simulink model "Target_Control_System"  (R2021b)
settings: Solver=FixedStepDiscrete  StartTime=0.0  StopTime=5  RelTol=1e-3
PreLoadFcn:
  | RTWConfigurationCB('preloadfcn', bdroot);
PostLoadFcn:
  | load('configuration/data_struct.mat');
  | load('configuration/fluxMaps_propMotor.mat');
  | load('configuration/parameterInit_PROP.mat');
  | load('configuration/parameterInit_PUMP.mat');
  | load('configuration/parameterInit_PITCH.mat');
  | load('configuration/parameterInit_TILT.mat');
  | %load('configuration/base_workspace_signal_definition.mat');
  | %load('resolvedatastores_to_baseworkspace_for_faster_simulation.mat');
model workspace (MAT data in the model file):
  SIMULATION_OPTIONS : Simulink.Parameter (value not decoded)
  TARGET_CODE_GEN : Simulink.Parameter (value not decoded)
  TCS_SAMPLE_FREQ_HZ : Simulink.Parameter (value not decoded)
symbols that are objects in the model workspace (value not decoded): TARGET_CODE_GEN, TCS_SAMPLE_FREQ_HZ
undefined symbols (not defined in the file): A_DQ_REF_LPF_INIT__PITCH, A_DQ_REF_LPF_INIT__PROP, A_DQ_REF_LPF_INIT__PUMP, A_DQ_REF_LPF_INIT__TILT, A_OBSERVER_CONFIDENCE_INIT__PITCH, A_OBSERVER_CONFIDENCE_INIT__PROP, A_OBSERVER_CONFIDENCE_INIT__PUMP, A_OBSERVER_CONFIDENCE_INIT__TILT, ACTUATOR_MAX_ANGLE_TRIP__PITCH, ACTUATOR_MIN_ANGLE_TRIP__PITCH, ACTUATOR_POS_SENSOR_INV_DIRECTION__PITCH, ACTUATOR_POS_SENSOR_INV_DIRECTION__TILT, ACTUATOR_POS_SENSOR_OFFSET__PITCH, ACTUATOR_POS_SENSOR_OFFSET__TILT, ADC_scaler1_baseaddr_TILT, ADC_SCALER_FLOAT_TO_FIXPOINT_EXPANSION, ANGLE_ELEC_FROM_SENSOR_OFFSET_INIT__PITCH, ANGLE_ELEC_FROM_SENSOR_OFFSET_INIT__PROP, ANGLE_ELEC_FROM_SENSOR_OFFSET_INIT__PUMP, ANGLE_ELEC_FROM_SENSOR_OFFSET_INIT__TILT, AUTO_CLEAR_FAULTS_ENABLED__PITCH, AUTO_CLEAR_FAULTS_ENABLED__PROP, AUTO_CLEAR_FAULTS_ENABLED__PUMP, AUTO_CLEAR_FAULTS_ENABLED__TILT, AUTO_CLEAR_FAULTS_WAIT_TICKS__PITCH, AUTO_CLEAR_FAULTS_WAIT_TICKS__PROP, AUTO_CLEAR_FAULTS_WAIT_TICKS__PUMP, AUTO_CLEAR_FAULTS_WAIT_TICKS__TILT, AUTO_I_ZERO_IDLE_TICKS__PITCH, AUTO_I_ZERO_IDLE_TICKS__PROP, AUTO_I_ZERO_IDLE_TICKS__PUMP, AUTO_I_ZERO_IDLE_TICKS__TILT, AUTO_I_ZERO_OFFSET_IDC_THRESHOLD__PITCH, AUTO_I_ZERO_OFFSET_IDC_THRESHOLD__PROP, AUTO_I_ZERO_OFFSET_IDC_THRESHOLD__PUMP, AUTO_I_ZERO_OFFSET_IDC_THRESHOLD__TILT, AUTO_I_ZERO_OFFSET_IPH_THRESHOLD__PITCH, AUTO_I_ZERO_OFFSET_IPH_THRESHOLD__PROP, AUTO_I_ZERO_OFFSET_IPH_THRESHOLD__PUMP, AUTO_I_ZERO_OFFSET_IPH_THRESHOLD__TILT, AUTO_SENSORLESS_SWITCHOVER_DISABLE_OMEGA, AUTO_SENSORLESS_SWITCHOVER_ENABLE_OMEGA, AUTO_SENSORLESS_SWITCHOVER_MIN_CONFIDENCE, AUXILIARY_PROTECTION_UNIT_BASEADDR__TILT, blanking_max_error_omega_INIT_PITCH, blanking_max_error_omega_INIT_TILT, blanking_max_error_position_INIT_PITCH, blanking_max_error_position_INIT_TILT, BRUTE_START_I_Q_REF_RAMP_SPEED__PITCH, BRUTE_START_I_Q_REF_RAMP_SPEED__PROP, BRUTE_START_I_Q_REF_RAMP_SPEED__PUMP, BRUTE_START_I_Q_REF_RAMP_SPEED__TILT, CONTROL_LOOP_DT_INIT__PITCH, CONTROL_LOOP_DT_INIT__PROP, CONTROL_LOOP_DT_INIT__PUMP, CONTROL_LOOP_DT_INIT__TILT, CORRECTION_FILTER_SCALE__PITCH, CORRECTION_FILTER_SCALE__PROP, CORRECTION_FILTER_SCALE__PUMP, CORRECTION_FILTER_SCALE__TILT ... (+458)
libraries: simulink x178, Reusables_Lib x24
(part 10 of 47)

== system Target_Control_System/Target_Control_System/InterruptFunction/pitchMotor_isrTask/currentController/Current Controller ==
  Enable : EnablePort
  Add1 : Sum
  Data Store Read1 : DataStoreRead  DataStoreName=oPitch  DataStoreElements=oPitch.oIsr_.oState_.fId_  IndexOptions=Index vector (dialog)  Indices=1  OutputSizes=1
  Data Store Read10 : DataStoreRead  DataStoreName=oPitch  DataStoreElements=oPitch.oIsr_.oParam_.oPiDataId_.oParameter_.fIntMax_  IndexOptions=Index vector (dialog)  Indices=1  OutputSizes=1
  Data Store Read11 : DataStoreRead  DataStoreName=oPitch  DataStoreElements=oPitch.oIsr_.oParam_.oPiDataId_.oParameter_.fLoopDt_  IndexOptions=Index vector (dialog)  Indices=1  OutputSizes=1
  Data Store Read13 : DataStoreRead  DataStoreName=oPitch  DataStoreElements=oPitch.oIsr_.oIn_.fIqRefRampOut_  IndexOptions=Index vector (dialog)  Indices=1  OutputSizes=1
  Data Store Read14 : DataStoreRead  DataStoreName=oPitch  DataStoreElements=oPitch.oIsr_.oIn_.fIdRefFractionOfIq_  IndexOptions=Index vector (dialog)  Indices=1  OutputSizes=1
  Data Store Read15 : DataStoreRead  DataStoreName=oPitch  DataStoreElements=oPitch.oIsr_.oState_.fIq_  IndexOptions=Index vector (dialog)  Indices=1  OutputSizes=1
  Data Store Read16 : DataStoreRead  DataStoreName=oPitch  DataStoreElements=oPitch.oIsr_.oParam_.oPiDataIq_.oParameter_.fKp_  IndexOptions=Index vector (dialog)  Indices=1  OutputSizes=1
  Data Store Read17 : DataStoreRead  DataStoreName=oPitch  DataStoreElements=oPitch.oIsr_.oIn_.fOneOverUdc_  IndexOptions=Index vector (dialog)  Indices=1  OutputSizes=1
  Data Store Read18 : DataStoreRead  DataStoreName=oPitch  DataStoreElements=oPitch.oIsr_.oParam_.oPiDataIq_.oParameter_.fKi_  IndexOptions=Index vector (dialog)  Indices=1  OutputSizes=1
  Data Store Read19 : DataStoreRead  DataStoreName=oPitch  DataStoreElements=oPitch.oIsr_.oParam_.oPiDataIq_.oParameter_.fLoopDt_  IndexOptions=Index vector (dialog)  Indices=1  OutputSizes=1
  Data Store Read2 : DataStoreRead  DataStoreName=oPitch  DataStoreElements=oPitch.oIsr_.oParam_.oPiDataId_.oParameter_.fKp_  IndexOptions=Index vector (dialog)  Indices=1  OutputSizes=1
  Data Store Read20 : DataStoreRead  DataStoreName=oPitch  DataStoreElements=oPitch.oIsr_.oParam_.oPiDataIq_.oParameter_.fIntMax_  IndexOptions=Index vector (dialog)  Indices=1  OutputSizes=1
  Data Store Read21 : DataStoreRead  DataStoreName=oPitch  DataStoreElements=oPitch.oIsr_.oParam_.oPiDataIq_.oParameter_.fOutMax_  IndexOptions=Index vector (dialog)  Indices=1  OutputSizes=1
  Data Store Read22 : DataStoreRead  DataStoreName=oPitch  DataStoreElements=oPitch.oIsr_.oParam_.oPiDataIq_.oParameter_.fIntMin_  IndexOptions=Index vector (dialog)  Indices=1  OutputSizes=1
  Data Store Read23 : DataStoreRead  DataStoreName=oPitch  DataStoreElements=oPitch.oIsr_.oParam_.oPiDataIq_.oParameter_.fOutMin_  IndexOptions=Index vector (dialog)  Indices=1  OutputSizes=1
  Data Store Read24 : DataStoreRead  DataStoreName=oPitch  DataStoreElements=oPitch.oIsr_.oState_.fFluxMainMagnitudeLpf_  IndexOptions=Index vector (dialog)  Indices=1  OutputSizes=1
  Data Store Read25 : DataStoreRead  DataStoreName=oPitch  DataStoreElements=oPitch.oIsr_.oIn_.fFluxFeedforwardGainRampOut_  IndexOptions=Index vector (dialog)  Indices=1  OutputSizes=1
  Data Store Read26 : DataStoreRead  DataStoreName=oPitch  DataStoreElements=oPitch.oIsr_.oIn_.fOneOverUdc_  IndexOptions=Index vector (dialog)  Indices=1  OutputSizes=1
  Data Store Read27 : DataStoreRead  DataStoreName=oPitch  DataStoreElements=oPitch.oIsr_.oParam_.fMaximumVoltageVectorLengthSquared_  IndexOptions=Index vector (dialog)  Indices=1  OutputSizes=1
  Data Store Read29 : DataStoreRead  DataStoreName=mdl_pitch_fOmegaE  IndexOptions=Index vector (dialog)  Indices=1  OutputSizes=1
  Data Store Read3 : DataStoreRead  DataStoreName=oPitch  DataStoreElements=oPitch.oIsr_.oParam_.oPiDataId_.oParameter_.fKi_  IndexOptions=Index vector (dialog)  Indices=1  OutputSizes=1
  Data Store Read30 : DataStoreRead  DataStoreName=oPitch  DataStoreElements=oPitch.oIsr_.oParam_.oPiDataIq_.fState_  IndexOptions=Index vector (dialog)  Indices=1  OutputSizes=1
  Data Store Read31 : DataStoreRead  DataStoreName=oPitch  DataStoreElements=oPitch.oIsr_.oIn_.fIdRefRampOut_  IndexOptions=Index vector (dialog)  Indices=1  OutputSizes=1
  Data Store Read5 : DataStoreRead  DataStoreName=oPitch  DataStoreElements=oPitch.oIsr_.oIn_.fOneOverUdc_  IndexOptions=Index vector (dialog)  Indices=1  OutputSizes=1
  Data Store Read6 : DataStoreRead  DataStoreName=oPitch  DataStoreElements=oPitch.oIsr_.oParam_.oPiDataId_.fState_  IndexOptions=Index vector (dialog)  Indices=1  OutputSizes=1
  Data Store Read7 : DataStoreRead  DataStoreName=oPitch  DataStoreElements=oPitch.oIsr_.oParam_.oPiDataId_.oParameter_.fOutMin_  IndexOptions=Index vector (dialog)  Indices=1  OutputSizes=1
  Data Store Read8 : DataStoreRead  DataStoreName=oPitch  DataStoreElements=oPitch.oIsr_.oParam_.oPiDataId_.oParameter_.fIntMin_  IndexOptions=Index vector (dialog)  Indices=1  OutputSizes=1
  Data Store Read9 : DataStoreRead  DataStoreName=oPitch  DataStoreElements=oPitch.oIsr_.oParam_.oPiDataId_.oParameter_.fOutMax_  IndexOptions=Index vector (dialog)  Indices=1  OutputSizes=1
  Data Store Write1 : DataStoreWrite  DataStoreName=oPitch  DataStoreElements=oPitch.oIsr_.oState_.fUqRef_  IndexOptions=Index vector (dialog)  Indices=1  OutputSizes=1
  Data Store Write2 : DataStoreWrite  DataStoreName=oPitch  DataStoreElements=oPitch.oIsr_.oState_.fUdRef_  IndexOptions=Index vector (dialog)  Indices=1  OutputSizes=1
  Data Store Write3 : DataStoreWrite  DataStoreName=oPitch  DataStoreElements=oPitch.oIsr_.oParam_.oPiDataIq_.fState_  IndexOptions=Index vector (dialog)  Indices=1  OutputSizes=1
  Data Store Write4 : DataStoreWrite  DataStoreName=oPitch  DataStoreElements=oPitch.oIsr_.oParam_.oPiDataId_.fState_  IndexOptions=Index vector (dialog)  Indices=1  OutputSizes=1
  Data Store Write5 : DataStoreWrite  DataStoreName=oPitch  DataStoreElements=oPitch.oIsr_.oState_.fUqRefPiContrib_  IndexOptions=Index vector (dialog)  Indices=1  OutputSizes=1
  Divide1 : Product  Inputs=**
  Flux Feed-forward : Subsystem
  Limit Voltage Vector : Subsystem
  PI Id Current Controller : Subsystem
  PI Iq Current Controller : Subsystem
  wires:
  Limit Voltage Vector/1(fUqRef_out) -> Data Store Write1/1
  Data Store Read11/1 -> PI Id Current Controller/6(fLoopDt)
  Data Store Read26/1 -> Flux Feed-forward/3(fOneOverUdc)
  PI Id Current Controller/1(fOutput) -> Limit Voltage Vector/1(fUdRef)
  Data Store Read27/1 -> Limit Voltage Vector/2(fMaximumVoltageVectorLengthSquared)
  Data Store Read17/1 -> PI Iq Current Controller/5(fScale)
  Data Store Read8/1 -> PI Id Current Controller/9(fIntMin)
  PI Id Current Controller/2(*fpState) -> Data Store Write4/1
  Data Store Read1/1 -> PI Id Current Controller/2(fActual)
  Data Store Read14/1 -> Divide1/1
  Data Store Read31/1 -> Add1/1
  Data Store Read21/1 -> PI Iq Current Controller/8(fOutMax)
  Data Store Read19/1 -> PI Iq Current Controller/6(fLoopDt)
  Data Store Read15/1 -> PI Iq Current Controller/2(fActual)
  Data Store Read18/1 -> PI Iq Current Controller/4(fKi)
  Data Store Read16/1 -> PI Iq Current Controller/3(fKp)
  Data Store Read10/1 -> PI Id Current Controller/7(fIntMax)
  PI Iq Current Controller/2(*fpState) -> Data Store Write3/1
  Add1/1 -> PI Id Current Controller/1(fTarget)
  Data Store Read23/1 -> PI Iq Current Controller/10(fOutMin)
  Data Store Read22/1 -> PI Iq Current Controller/9(fIntMin)
  Data Store Read7/1 -> PI Id Current Controller/10(fOutMin)
  Data Store Read25/1 -> Flux Feed-forward/2(fFluxFeedforwardGainRampOut)
  Divide1/1 -> Add1/2
  Data Store Read24/1 -> Flux Feed-forward/1(fFluxMainMagnitudeLpf)
  Data Store Read29/1 -> Flux Feed-forward/5(mdl_tilt_fOmegaE)
  Limit Voltage Vector/2(fUdRef_out) -> Data Store Write2/1
  Flux Feed-forward/1(fUqRef) -> Limit Voltage Vector/3(fUqRef)
  Data Store Read20/1 -> PI Iq Current Controller/7(fIntMax)
  Data Store Read9/1 -> PI Id Current Controller/8(fOutMax)
  Data Store Read5/1 -> PI Id Current Controller/5(fScale)
  Data Store Read2/1 -> PI Id Current Controller/3(fKp)
  Data Store Read3/1 -> PI Id Current Controller/4(fKi)
  Data Store Read30/1 -> PI Iq Current Controller/11(fState)
  Data Store Read6/1 -> PI Id Current Controller/11(fState)
  PI Iq Current Controller/1(fOutput) -> Flux Feed-forward/4(fUqRefPiContrib), Data Store Write5/1
  Data Store Read13/1 -> PI Iq Current Controller/1(fTarget), Divide1/2

== system Target_Control_System/Target_Control_System/InterruptFunction/pitchMotor_isrTask/dqTransform/DQ Transform ==
  fIAlpha : Inport
  fIBeta : Inport  Port=2
  Data Store Read1 : DataStoreRead  DataStoreName=mdl_pitch_fFluxMasterAngle_cos_  IndexOptions=Index vector (dialog)  Indices=1  OutputSizes=1
  Data Store Read2 : DataStoreRead  DataStoreName=mdl_pitch_fFluxMasterAngle_sin_  IndexOptions=Index vector (dialog)  Indices=1  OutputSizes=1
  Mux2 : Mux  Inputs=2
  Mux5 : Mux
  Square Root Sum : Fcn  Expr=sqrt((u(1)*u(1))+(u(2)*u(2)))
  fId_ = fCosTerm*opState->fIAlpha_ + fSinTerm*opState->fIBeta_ : Fcn  Expr=u(4)*u(1)+u(3)*u(2)
  fIq_ = fCosTerm*opState->fIBeta_ - fSinTerm*opState->fIAlpha_ : Fcn  Expr=u(4)*u(2)-u(3)*u(1)
  fId : Outport
  fIq : Outport  Port=2
  fIPhaseMagnitude : Outport  Port=3
  wires:
  Data Store Read1/1 -> Mux5/4
  Data Store Read2/1 -> Mux5/3
  fIBeta/1 -> Mux5/2
  fIAlpha/1 -> Mux5/1
  Mux2/1 -> Square Root Sum/1
  fIq_ = fCosTerm*opState->fIBeta_ - fSinTerm*opState->fIAlpha_/1 -> Mux2/2, fIq/1
  Mux5/1 -> fId_ = fCosTerm*opState->fIAlpha_ + fSinTerm*opState->fIBeta_/1, fIq_ = fCosTerm*opState->fIBeta_ - fSinTerm*opState->fIAlpha_/1
  fId_ = fCosTerm*opState->fIAlpha_ + fSinTerm*opState->fIBeta_/1 -> Mux2/1, fId/1
  Square Root Sum/1 -> fIPhaseMagnitude/1

== system Target_Control_System/Target_Control_System/InterruptFunction/pitchMotor_isrTask/dqTransform/Torque_Estimation_Pitch ==
  fPolePairs : Inport
  fFluxMainMagnitudeLpf : Inport  Port=2
  fIq : Inport  Port=3
  Divide : Product  Inputs=***
  Gain : Gain  Gain=1.5
  fTEstimate : Outport
  wires:
  Gain/1 -> fTEstimate/1
  fPolePairs/1 -> Divide/1
  fFluxMainMagnitudeLpf/1 -> Divide/2
  fIq/1 -> Divide/3
  Divide/1 -> Gain/1

== system Target_Control_System/Target_Control_System/InterruptFunction/pitchMotor_isrTask/fluxAngleCalculations/Advance Forced Angle ==
  Input : Inport
  Integrator with Angle Wrapper : Subsystem
  Integrator with Angle Wrapper_OLD : Subsystem  Commented=on
  Output : Outport
  wires:
  Integrator with Angle Wrapper/1(Angle) -> Output/1
  Input/1 -> Integrator with Angle Wrapper/1(Omega)

== system Target_Control_System/Target_Control_System/InterruptFunction/pitchMotor_isrTask/fluxAngleCalculations/Back Rotation ==
  fFluxMasterAngleOffsetRampOut : Inport
  fFluxMasterAngle : Inport  Port=2
  Add6 : Sum
  Angle Clip : Subsystem
  fFluxMasterAngleBkwd : Outport
  wires:
  Angle Clip/1(Angle_Out) -> fFluxMasterAngleBkwd/1
  fFluxMasterAngle/1 -> Add6/2
  Add6/1 -> Angle Clip/1(Angle_In)
  fFluxMasterAngleOffsetRampOut/1 -> Add6/1

== system Target_Control_System/Target_Control_System/InterruptFunction/pitchMotor_isrTask/fluxAngleCalculations/ModelSource ==
  note: 1) Add Subsystem or Model blocks as valid variant choices.
      | 2) You cannot connect blocks at this level. At simulation, connectivity is automatically
      | determined, based on the active variant and port name matching.
  DoNotIncludeCustomCode : Subsystem  TreatAsAtomicUnit=on  VariantControl=TARGET_CODE_GEN == 0
  IncludeCustomCode : Subsystem  TreatAsAtomicUnit=on  VariantControl=(default)

== system Target_Control_System/Target_Control_System/InterruptFunction/pitchMotor_isrTask/fluxAngleCalculations/Not forced Angle ==
  iUseSensorAngle : Inport
  fAngleElecFromPosSensor : Inport  Port=2
  fFluxMainAngleRaw2 : Inport  Port=3
  fOmegaElecFromPosSensor : Inport  Port=4
  fOmegaEObserverLpf2 : Inport  Port=5
  fFluxMasterAngleForced2closedSmoothingRampOut : Inport  Port=6
  Add1 : Sum
  Angle Clip : Subsystem
  Equal1 : RelationalOperator  Operator===  OutDataTypeStr=boolean  RndMeth=Simplest
  Equal3 : RelationalOperator  Operator=~=  OutDataTypeStr=boolean  RndMeth=Simplest
  One1 : Constant  OutDataTypeStr=int32  SampleTime=-1
  Switch1 : Switch  Criteria=u2 > Threshold  Threshold=0.5
  Switch3 : Switch  Criteria=u2 > Threshold  Threshold=0.5
  Switch4 : Switch  Criteria=u2 > Threshold  Threshold=0.5
  Zero2 : Constant  Value=0  OutDataTypeStr=single  SampleTime=-1
  fFluxMasterAngle : Outport
  fOmegaE : Outport  Port=2
  wires:
  Switch1/1 -> fFluxMasterAngle/1
  fOmegaEObserverLpf2/1 -> Switch4/3
  fOmegaElecFromPosSensor/1 -> Switch4/1
  fFluxMainAngleRaw2/1 -> Switch3/3
  fAngleElecFromPosSensor/1 -> Switch3/1
  iUseSensorAngle/1 -> Equal1/2
  Angle Clip/1(Angle_Out) -> Switch1/1
  Switch3/1 -> Switch1/3, Add1/2  "fFluxMasterAngle"
  One1/1 -> Equal1/1
  Zero2/1 -> Equal3/1
  Add1/1 -> Angle Clip/1(Angle_In)
  fFluxMasterAngleForced2closedSmoothingRampOut/1 -> Add1/1, Equal3/2
  Equal3/1 -> Switch1/2
  Switch4/1 -> fOmegaE/1
  Equal1/1 -> Switch3/2, Switch4/2

== system Target_Control_System/Target_Control_System/InterruptFunction/pitchMotor_isrTask/fluxAngleCalculations/vsincos() ==
  fFluxMasterAngleBkwd : Inport
  fFluxMasterAngle : Inport  Port=2
  Enable : EnablePort
  Cos2 : Trigonometry  Operator=cos
  Cos3 : Trigonometry  Operator=cos
  Data Store Write1 : DataStoreWrite  DataStoreName=mdl_pitch_fFluxMasterAngle_cos_  IndexOptions=Index vector (dialog)  Indices=1  OutputSizes=1
  Data Store Write2 : DataStoreWrite  DataStoreName=mdl_pitch_fFluxMasterAngle_sin_  IndexOptions=Index vector (dialog)  Indices=1  OutputSizes=1
  Data Store Write7 : DataStoreWrite  DataStoreName=mdl_pitch_fFluxMasterAngleBkwd_sin_  IndexOptions=Index vector (dialog)  Indices=1  OutputSizes=1
  Data Store Write8 : DataStoreWrite  DataStoreName=mdl_pitch_fFluxMasterAngleBkwd_cos_  IndexOptions=Index vector (dialog)  Indices=1  OutputSizes=1
  Sin2 : Trigonometry
  Sin3 : Trigonometry
  wires:
  fFluxMasterAngle/1 -> Sin2/1, Cos2/1
  fFluxMasterAngleBkwd/1 -> Sin3/1, Cos3/1
  Sin2/1 -> Data Store Write2/1
  Cos2/1 -> Data Store Write1/1
  Sin3/1 -> Data Store Write7/1
  Cos3/1 -> Data Store Write8/1

== system Target_Control_System/Target_Control_System/InterruptFunction/pitchMotor_isrTask/fluxObserver/Calculate Coil Flux + Bleeder ==
  fControlLoopDt : Inport
  fKFluxBleeder : Inport  Port=2
  fUAlpha : Inport  Port=3
  fUBeta : Inport  Port=4
  Discrete-Time Integrator12 : DiscreteIntegrator  SampleTime=-1  OutDataTypeStr=single  UpperSaturationLimit=2*pi*100  LowerSaturationLimit=-2*pi*100  ICPrevOutput=DiscIntNeverNeededParam  ICPrevScaledInput=DiscIntNeverNeededParam
  Discrete-Time Integrator13 : DiscreteIntegrator  SampleTime=-1  OutDataTypeStr=single  UpperSaturationLimit=2*pi*100  LowerSaturationLimit=-2*pi*100  ICPrevOutput=DiscIntNeverNeededParam  ICPrevScaledInput=DiscIntNeverNeededParam
  Product2 : Product  Inputs=3
  Product3 : Product  Inputs=3
  Sum25 : Sum  Inputs=+-|
  Sum26 : Sum  Inputs=|-+
  fFluxCoilAlpha : Outport
  fFluxCoilBeta : Outport  Port=2
  wires:
  fUBeta/1 -> Discrete-Time Integrator13/1
  fUAlpha/1 -> Discrete-Time Integrator12/1
  fKFluxBleeder/1 -> Product3/1, Product2/3
  Product2/1 -> Sum25/2
  Sum25/1 -> fFluxCoilAlpha/1
  Sum26/1 -> fFluxCoilBeta/1
  Product3/1 -> Sum26/1
  fControlLoopDt/1 -> Product2/2, Product3/2
  Discrete-Time Integrator12/1 -> Sum25/1, Product2/1  "fFluxCoilAlpha"
  Discrete-Time Integrator13/1 -> Product3/3, Sum26/2  "fFluxCoilBeta"

== system Target_Control_System/Target_Control_System/InterruptFunction/pitchMotor_isrTask/fluxObserver/Calculate Main Flux + LPF ==
  fIAlphaLocal : Inport
  fIBetaLocal : Inport  Port=2
  fLsPhase : Inport  Port=3
  fFluxCoilAlpha : Inport  Port=4
  fFluxCoilBeta : Inport  Port=5
  Constant3 : Constant  Value=8*2*pi  OutDataTypeStr=single  SampleTime=-1
  Data Store Read33 : DataStoreRead  Commented=on  DataStoreName=oPitch  DataStoreElements=oPitch.oIsr_.oParam_.fAFluxMagnitude_  IndexOptions=Index vector (dialog)  Indices=1  OutputSizes=1
  Discrete-Time Integrator5 : DiscreteIntegrator  SampleTime=-1  OutDataTypeStr=single  UpperSaturationLimit=2*pi*100  LowerSaturationLimit=-2*pi*100  ICPrevOutput=DiscIntNeverNeededParam  ICPrevScaledInput=DiscIntNeverNeededParam
  Divide10 : Product  Inputs=**
  Divide8 : Product  Inputs=**
  Divide9 : Product  Inputs=**
  Mux : Mux  Inputs=2
  Sum27 : Sum  Inputs=-+|
  Sum28 : Sum  Inputs=-+|
  Sum29 : Sum  Inputs=-+|
  sqrt root sum1 : Fcn  Expr=sqrt((u(1)*u(1))+(u(2)*u(2)))
  fFluxMainAlpha : Outport
  fFluxMainBeta : Outport  Port=2
  fFluxMainMagnitude : Outport  Port=3
  fFluxMainMagnitudeLpf : Outport  Port=4
  wires:
  fFluxCoilBeta/1 -> Sum28/2
  fFluxCoilAlpha/1 -> Sum27/2
  fIBetaLocal/1 -> Divide9/1
  fIAlphaLocal/1 -> Divide8/1
  Sum28/1 -> Mux/2, fFluxMainBeta/1  "fFluxMainBeta"
  Divide10/1 -> Discrete-Time Integrator5/1
  Sum27/1 -> Mux/1, fFluxMainAlpha/1  "fFluxMainAlpha"
  fLsPhase/1 -> Divide8/2, Divide9/2
  sqrt root sum1/1 -> Sum29/2, fFluxMainMagnitude/1
  Constant3/1 -> Divide10/2
  Mux/1 -> sqrt root sum1/1
  Sum29/1 -> Divide10/1
  Divide8/1 -> Sum27/1
  Discrete-Time Integrator5/1 -> Sum29/1, fFluxMainMagnitudeLpf/1  "fFluxMainMagnitudeLpf"
  Divide9/1 -> Sum28/1

== system Target_Control_System/Target_Control_System/InterruptFunction/pitchMotor_isrTask/fluxObserver/Fast PLL ==
  fluxAngle_sin : Inport
  fluxAngle_cos : Inport  Port=2
  fFluxMainAlpha : Inport  Port=3
  fFluxMainBeta : Inport  Port=4
  fObserverLoopFilterBandwidthHz : Inport  Port=5
  oPiDataPll2_.fState : Inport  Port=6
  oPiDataPll2_.oParameter : Inport  Port=7
  " " : Constant  OutDataTypeStr=single  SampleTime=-1
  Atan2 : Trigonometry  Operator=atan2
  Constant4 : Constant  Value=2*pi  OutDataTypeStr=single  SampleTime=-1
  Data Store Read : DataStoreRead  Commented=on  DataStoreName=oPitch  DataStoreElements=oPitch.oIsr_.oParam_.fALoopfilter2_  IndexOptions=Index vector (dialog)  Indices=1  OutputSizes=1
  Data Store Read4 : DataStoreRead  Commented=on  DataStoreName=oPitch  DataStoreElements=oPitch.oIsr_.oParam_.fAOmegaFilter2_  IndexOptions=Index vector (dialog)  Indices=1  OutputSizes=1
  Demux : Demux  Outputs=7
  Discrete-Time Integrator : DiscreteIntegrator  SampleTime=-1  ICPrevOutput=DiscIntNeverNeededParam  ICPrevScaledInput=DiscIntNeverNeededParam
  Discrete-Time Integrator11 : DiscreteIntegrator  SampleTime=-1  OutDataTypeStr=single  ICPrevOutput=DiscIntNeverNeededParam  ICPrevScaledInput=DiscIntNeverNeededParam
  Fcn : Fcn  Expr=u(1)*u(4)+u(2)*u(3)
  Fcn3 : Fcn  Expr=-u(1)*u(3)+u(2)*u(4)
  Mux13 : Mux
  Product17 : Product  Inputs=3
  Q-axis PLL_target : Constant  Value=0  OutDataTypeStr=single  SampleTime=-1
  Sum1 : Sum  Inputs=-+|
  Sum2 : Sum  Inputs=-+|
  fAOmegaFilter2_ : Gain  Gain=100.0*2*pi
  piControllerStep_fOmegaE_pitch : Subsystem
  fAtan2loopfilter2Out : Outport
  oPiDataPll2_.fState* : Outport  Port=2
  fOmegaEObserverRaw2 : Outport  Port=3
  fOmegaEObserverLpf2 : Outport  Port=4
  wires:
  oPiDataPll2_.oParameter/1 -> Demux/1
  oPiDataPll2_.fState/1 -> piControllerStep_fOmegaE_pitch/11(fState)
  Demux/7 -> piControllerStep_fOmegaE_pitch/10(fOutMin)
  Demux/6 -> piControllerStep_fOmegaE_pitch/9(fIntMin)
  Demux/5 -> piControllerStep_fOmegaE_pitch/8(fOutMax)
  Demux/4 -> piControllerStep_fOmegaE_pitch/7(fIntMax)
  Demux/3 -> piControllerStep_fOmegaE_pitch/6(fLoopDt)
  Demux/2 -> piControllerStep_fOmegaE_pitch/5(fKi)
  Demux/1 -> piControllerStep_fOmegaE_pitch/4(fKp)
  fObserverLoopFilterBandwidthHz/1 -> Product17/2
  fFluxMainAlpha/1 -> Mux13/1
  fFluxMainBeta/1 -> Mux13/2
  Sum1/1 -> Product17/1
  Atan2/1 -> Sum1/2  "fAtan2output"
  Product17/1 -> Discrete-Time Integrator/1
  Fcn3/1 -> Atan2/1  "fPLLQ"
  " "/1 -> piControllerStep_fOmegaE_pitch/1(fScale)
  Sum2/1 -> fAOmegaFilter2_/1
  fAOmegaFilter2_/1 -> Discrete-Time Integrator11/1
  Mux13/1 -> Fcn/1, Fcn3/1
  Fcn/1 -> Atan2/2  "fPLLD"
  piControllerStep_fOmegaE_pitch/2(*fpState) -> oPiDataPll2_.fState*/1
  Discrete-Time Integrator/1 -> piControllerStep_fOmegaE_pitch/3(fTarget), Sum1/1, fAtan2loopfilter2Out/1  "fAtan2loopfilter2Out_"
  fluxAngle_cos/1 -> Mux13/4
  Constant4/1 -> Product17/3
  Discrete-Time Integrator11/1 -> fOmegaEObserverLpf2/1, Sum2/1  "fOmegaEObserverLpf2_"
  piControllerStep_fOmegaE_pitch/1(fOutput) -> Sum2/2, fOmegaEObserverRaw2/1
  Q-axis PLL_target/1 -> piControllerStep_fOmegaE_pitch/2(fActual)
  fluxAngle_sin/1 -> Mux13/3

== system Target_Control_System/Target_Control_System/InterruptFunction/pitchMotor_isrTask/fluxObserver/HPF Currents ==
  fIAlpha : Inport
  fIBeta : Inport  Port=2
  Constant2 : Constant  Value=15*2*pi  OutDataTypeStr=single  SampleTime=-1
  Data Store Read24 : DataStoreRead  Commented=on  DataStoreName=oPitch  DataStoreElements=oPitch.oIsr_.oParam_.fALpf4hpfDcBlocking_  IndexOptions=Index vector (dialog)  Indices=1  OutputSizes=1
  Discrete-Time Integrator3 : DiscreteIntegrator  SampleTime=-1  OutDataTypeStr=single  UpperSaturationLimit=2*pi*100  LowerSaturationLimit=-2*pi*100  ICPrevOutput=DiscIntNeverNeededParam  ICPrevScaledInput=DiscIntNeverNeededParam
  Discrete-Time Integrator4 : DiscreteIntegrator  SampleTime=-1  OutDataTypeStr=single  UpperSaturationLimit=2*pi*100  LowerSaturationLimit=-2*pi*100  ICPrevOutput=DiscIntNeverNeededParam  ICPrevScaledInput=DiscIntNeverNeededParam
  Divide2 : Product  Inputs=**
  Divide3 : Product  Inputs=**
  Sum13 : Sum  Inputs=-+|
  Sum14 : Sum  Inputs=|-+
  Sum15 : Sum  Inputs=-+|
  Sum16 : Sum  Inputs=|-+
  fIAlphaLpf4hpf : Outport
  fIBetaLpf4hpf : Outport  Port=2
  fIAlphaLocal : Outport  Port=3
  fIBetaLocal : Outport  Port=4
  wires:
  Discrete-Time Integrator3/1 -> Sum16/1, fIBetaLpf4hpf/1, Sum15/1  "fIBetaLpf4hpf_"
  Sum13/1 -> Divide2/2
  Divide3/1 -> Discrete-Time Integrator3/1
  Discrete-Time Integrator4/1 -> Sum13/1, fIAlphaLpf4hpf/1, Sum14/1  "fIAlphaLpf4hpf_"
  fIAlpha/1 -> Sum13/2, Sum14/2
  Sum15/1 -> Divide3/2
  Divide2/1 -> Discrete-Time Integrator4/1
  Constant2/1 -> Divide2/1, Divide3/1
  fIBeta/1 -> Sum16/2, Sum15/2
  Sum16/1 -> fIBetaLocal/1  "fIBetaLocal"
  Sum14/1 -> fIAlphaLocal/1  "fIAlphaLocal"

== system Target_Control_System/Target_Control_System/InterruptFunction/pitchMotor_isrTask/fluxObserver/HPF Voltages ==
  fUAlpha : Inport
  fUBeta : Inport  Port=2
  Constant : Constant  Value=15*2*pi  OutDataTypeStr=single  SampleTime=-1
  Data Store Read26 : DataStoreRead  Commented=on  DataStoreName=oPitch  DataStoreElements=oPitch.oIsr_.oParam_.fALpf4hpfDcBlocking_  IndexOptions=Index vector (dialog)  Indices=1  OutputSizes=1
  Discrete-Time Integrator1 : DiscreteIntegrator  SampleTime=-1  OutDataTypeStr=single  UpperSaturationLimit=2*pi*100  LowerSaturationLimit=-2*pi*100  ICPrevOutput=DiscIntNeverNeededParam  ICPrevScaledInput=DiscIntNeverNeededParam
  Discrete-Time Integrator2 : DiscreteIntegrator  SampleTime=-1  OutDataTypeStr=single  UpperSaturationLimit=2*pi*100  LowerSaturationLimit=-2*pi*100  ICPrevOutput=DiscIntNeverNeededParam  ICPrevScaledInput=DiscIntNeverNeededParam
  Divide6 : Product  Inputs=**
  Divide7 : Product  Inputs=**
  Sum21 : Sum  Inputs=-+|
  Sum22 : Sum  Inputs=|-+
  Sum23 : Sum  Inputs=-+|
  Sum24 : Sum  Inputs=|-+
  fUAlphaLpf4hpf : Outport
  fUBetaLpf4hpf : Outport  Port=2
  fUAlpha_out : Outport  Port=3
  fUBeta_out : Outport  Port=4
  wires:
  Divide6/1 -> Discrete-Time Integrator2/1
  Sum24/1 -> fUBeta_out/1  "fUBetaLpf"
  Discrete-Time Integrator1/1 -> Sum24/1, fUBetaLpf4hpf/1, Sum23/1  "fUBetaLpf4hpf_"
  Sum21/1 -> Divide6/2
  Discrete-Time Integrator2/1 -> Sum21/1, Sum22/1, fUAlphaLpf4hpf/1  "fUAlphaLpf4hpf_"
  Divide7/1 -> Discrete-Time Integrator1/1
  fUBeta/1 -> Sum23/2, Sum24/2
  Sum23/1 -> Divide7/2
  fUAlpha/1 -> Sum21/2, Sum22/2
  Constant/1 -> Divide6/1, Divide7/1
  Sum22/1 -> fUAlpha_out/1  "fUAlphaLpf"

== system Target_Control_System/Target_Control_System/InterruptFunction/pitchMotor_isrTask/fluxObserver/Subtract Resistive Voltage Drop ==
  fIAlphaLocal : Inport
  fIBetaLocal : Inport  Port=2
  fRsPhase : Inport  Port=3
  fUAlpha : Inport  Port=4
  fUBeta : Inport  Port=5
  Divide4 : Product  Inputs=**
  Divide5 : Product  Inputs=**
  Sum17 : Sum  Inputs=-+|
  Sum20 : Sum  Inputs=-+|
  fUAlpha_out : Outport
  fUBeta_out : Outport  Port=2
  wires:
  Divide5/1 -> Sum17/1
  fUBeta/1 -> Sum17/2
  fUAlpha/1 -> Sum20/2
  fIBetaLocal/1 -> Divide5/2
  Sum17/1 -> fUBeta_out/1  "fUBetaMinusRs"
  Sum20/1 -> fUAlpha_out/1  "fUAlphaMinusRs"
  Divide4/1 -> Sum20/1
  fRsPhase/1 -> Divide4/1, Divide5/1
  fIAlphaLocal/1 -> Divide4/2

== system Target_Control_System/Target_Control_System/InterruptFunction/pitchMotor_isrTask/fluxObserver/Ultra Raw Angle ==
  fFluxMainAlpha : Inport
  fFluxMainBeta : Inport  Port=2
  Atan2 : Trigonometry  Operator=atan2
  fFluxMainAngleUltraRaw : Outport
  wires:
  fFluxMainBeta/1 -> Atan2/1
  fFluxMainAlpha/1 -> Atan2/2
  Atan2/1 -> fFluxMainAngleUltraRaw/1

== system Target_Control_System/Target_Control_System/InterruptFunction/pitchMotor_isrTask/fluxObserver/Voltage Vector Rotation ==
  UphFilterDelayAngleRad_sin : Inport
  UphFilterDelayAngleRad_cos : Inport  Port=2
  fUphFilterAmplitudeRatio : Inport  Port=3
  uiUphFilterCorrectionEnabled : Inport  Port=4
  fUAlpha : Inport  Port=5
  fUBeta : Inport  Port=6
  Demux : Demux  Outputs=2
  Divide1 : Product  Inputs=*/
  Fcn1 : Fcn  Expr=u(1)*u(4)-u(2)*u(3)
  Fcn2 : Fcn  Expr=u(1)*u(3)+u(2)*u(4)
  Mux2 : Mux  Inputs=2
  Mux7 : Mux  Inputs=2
  Mux8 : Mux  Inputs=3
  Switch5 : Switch  Criteria=u2 > Threshold  Threshold=0.5
  fUAlpha_out : Outport
  fUBeta_out : Outport  Port=2
  wires:
  fUBeta/1 -> Mux2/2
  fUAlpha/1 -> Mux2/1
  uiUphFilterCorrectionEnabled/1 -> Switch5/2
  fUphFilterAmplitudeRatio/1 -> Divide1/2
  Demux/2 -> fUBeta_out/1
  Demux/1 -> fUAlpha_out/1
  Switch5/1 -> Demux/1
  Mux2/1 -> Mux8/1, Switch5/3
  UphFilterDelayAngleRad_cos/1 -> Mux8/3
  UphFilterDelayAngleRad_sin/1 -> Mux8/2
  Divide1/1 -> Switch5/1
  Fcn1/1 -> Mux7/1  "fUAlpha_"
  Mux7/1 -> Divide1/1
  Fcn2/1 -> Mux7/2  "fUBeta_"
  Mux8/1 -> Fcn1/1, Fcn2/1

== system Target_Control_System/Target_Control_System/InterruptFunction/pitchMotor_isrTask/pwmGeneration/Subsystem ==
  Enable : EnablePort
  ABC to DQ : Subsystem
  Calculate Duty Cycles : Subsystem
  Constant : Constant  OutDataTypeStr=int32  SampleTime=-1
  Constant1 : Constant  Commented=on  OutDataTypeStr=uint32  SampleTime=-1
  Data Store Read1 : DataStoreRead  DataStoreName=mdl_pitch_fFluxMasterAngleBkwd_cos_  IndexOptions=Index vector (dialog)  Indices=1  OutputSizes=1
  Data Store Read11 : DataStoreRead  DataStoreName=oPitch  DataStoreElements=oPitch.oIsr_.oState_.fUdRef_  IndexOptions=Index vector (dialog)  Indices=1  OutputSizes=1
  Data Store Read12 : DataStoreRead  DataStoreName=oPitch  DataStoreElements=oPitch.oIsr_.oState_.fUqRef_  IndexOptions=Index vector (dialog)  Indices=1  OutputSizes=1
  Data Store Read13 : DataStoreRead  DataStoreName=mdl_pitch_fFluxMasterAngleBkwd_sin_  IndexOptions=Index vector (dialog)  Indices=1  OutputSizes=1
  Data Store Read2 : DataStoreRead  DataStoreName=oPitch  DataStoreElements=oPitch.oIsr_.oParam_.iInverseDirection_  IndexOptions=Index vector (dialog)  Indices=1  OutputSizes=1
  Data Store Read3 : DataStoreRead  DataStoreName=oPitch  DataStoreElements=oPitch.oIsr_.oParam_.fPwmPeriodTicksFloat_  IndexOptions=Index vector (dialog)  Indices=1  OutputSizes=1
  Data Store Read4 : DataStoreRead  DataStoreName=oPitch  DataStoreElements=oPitch.oIsr_.oParam_.fHalfPositiveDuty_  IndexOptions=Index vector (dialog)  Indices=1  OutputSizes=1
  Data Store Read5 : DataStoreRead  DataStoreName=oPitch  DataStoreElements=oPitch.oIsr_.oParam_.fMaximumDuty_  IndexOptions=Index vector (dialog)  Indices=1  OutputSizes=1
  Data Store Write1 : DataStoreWrite  DataStoreName=oPitch  DataStoreElements=oPitch.oIsr_.oOut_.uiPwmDutyTicksA_  IndexOptions=Index vector (dialog)  Indices=1  OutputSizes=1
  Data Store Write2 : DataStoreWrite  DataStoreName=oPitch  DataStoreElements=oPitch.oIsr_.oOut_.uiPwmDutyTicksB_  IndexOptions=Index vector (dialog)  Indices=1  OutputSizes=1
  Data Store Write3 : DataStoreWrite  DataStoreName=oPitch  DataStoreElements=oPitch.oIsr_.oOut_.uiPwmDutyTicksC_  IndexOptions=Index vector (dialog)  Indices=1  OutputSizes=1
  Data Store Write4 : DataStoreWrite  DataStoreName=oPitch  DataStoreElements=oPitch.oIsr_.oState_.iPwmUpdated_  IndexOptions=Index vector (dialog)  Indices=1  OutputSizes=1
  Data Store Write5 : DataStoreWrite  Commented=on  DataStoreName=oPitch  DataStoreElements=oPitch.oIsr_.oOut_.uiPwmSetByIsr_  IndexOptions=Index vector (dialog)  Indices=1  OutputSizes=1
  Zero sequence injection : Subsystem
  wires:
  Data Store Read11/1 -> ABC to DQ/2(UdRef)  "UdRef"
  Data Store Read12/1 -> ABC to DQ/3(UqRef)  "UqRef"
  Calculate Duty Cycles/2(uiPwmDutyTicksB) -> Data Store Write2/1
  Calculate Duty Cycles/3(uiPwmDutyTicksC) -> Data Store Write3/1
  Calculate Duty Cycles/1(uiPwmDutyTicksA) -> Data Store Write1/1
  Data Store Read4/1 -> Calculate Duty Cycles/5(fHalfPositiveDuty)
  Data Store Read3/1 -> Calculate Duty Cycles/6(fPwmPeriodTicksFloat)
  Zero sequence injection/3(fUcRef) -> Calculate Duty Cycles/3(fUcRef)
  Data Store Read5/1 -> Calculate Duty Cycles/4(fMaximumDuty)
  ABC to DQ/1(U_abc) -> Zero sequence injection/1(U_abc)
  Zero sequence injection/1(fUaRef) -> Calculate Duty Cycles/1(fUaRef)
  Data Store Read1/1 -> ABC to DQ/5(fFluxMasterAngleBkwd_cos)
  Zero sequence injection/2(fUbRef) -> Calculate Duty Cycles/2(fUbRef)
  Data Store Read2/1 -> ABC to DQ/1(iInverseDirection)
  Data Store Read13/1 -> ABC to DQ/4(fFluxMasterAngleBkwd_sin)
  Constant1/1 -> Data Store Write5/1
  Constant/1 -> Data Store Write4/1

== system Target_Control_System/Target_Control_System/InterruptFunction/pitchMotor_setPwm/ModelSourceFPGAPitch/DoNotIncludeCustomCode ==

== system Target_Control_System/Target_Control_System/InterruptFunction/pitchMotor_setPwm/ModelSourceFPGAPitch/IncludeCustomCode ==
  System Update : Subsystem  mask(System Update){ShowInLibBrowser=0}
      mask prompts: ShowInLibBrowser "Simulink:masks:CustCodeMaskParam1_MP"
      settings: CopyFcn=cccopyfcn(gcb)  OpenFcn=ccopenfcn('System Update Function')
      mask Help: eval('feval(''rtwprivate'',''rtwhelpview'',''rtw_sys_update_block'')');
      mask DialogControl ShowInLibBrowser Prompt: Mask Parameter 1:
      mask Display: disp('System\nUpdate');

== system Target_Control_System/Target_Control_System/InterruptFunction/propMotor_IsrSchedule/Isr_Variant/CodeGen_IsrEnable ==
  Compare To Zero : simulink/Logic and Bit Operations/Compare To Zero  relop=>  OutDataTypeStr=boolean
  Data Store Read1 : DataStoreRead  DataStoreName=fpga_uiPWMInterruptCount_  IndexOptions=Index vector (dialog)  Indices=1  OutputSizes=1
  manageSmallInverterCounter : Subsystem  Priority=5  TreatAsAtomicUnit=on
  IsrCall : Outport
  wires:
  manageSmallInverterCounter/1(IsrEnable) -> IsrCall/1
  Data Store Read1/1 -> Compare To Zero/1
  Compare To Zero/1 -> manageSmallInverterCounter/Trigger

== system Target_Control_System/Target_Control_System/InterruptFunction/propMotor_IsrSchedule/Isr_Variant/Simulation_IsrEnable ==
  Add : Sum
  Data Store Read : DataStoreRead  DataStoreName=mdl_suiIsrSmallInvCounter_  IndexOptions=Index vector (dialog)  Indices=1  OutputSizes=1
  Data Store Read1 : DataStoreRead  DataStoreName=fpga_uiPWMInterruptCount_  IndexOptions=Index vector (dialog)  Indices=1  OutputSizes=1
  Data Store Write1 : DataStoreWrite  DataStoreName=mdl_suiIsrSmallInvCounter_  IndexOptions=Index vector (dialog)  Indices=1  OutputSizes=1
  Function-Call Generator : simulink/Ports & Subsystems/Function-Call Generator  sample_time=-1  numberOfIterations=1  DisallowWideOutput=off
  Switch : Switch  Criteria=u2 > Threshold  Threshold=3
  constant1 : Constant  OutDataTypeStr=uint32  SampleTime=-1
  constant2 : Constant  Value=0  OutDataTypeStr=uint32  SampleTime=-1
  IsrCall : Outport
  wires:
  Add/1 -> Switch/2, Switch/3
  constant1/1 -> Add/2
  Function-Call Generator/1 -> IsrCall/1
  Data Store Read/1 -> Add/1
  constant2/1 -> Switch/1
  Switch/1 -> Data Store Write1/1

== system Target_Control_System/Target_Control_System/InterruptFunction/propMotor_isrTask/abcToAlphaBeta/Integrator with Angle Wrapper ==
  Omega : Inport
  Add : Sum  Commented=on  Inputs=+-
  Add1 : Sum  Commented=on
  Add5 : Sum
  Add6 : Sum  Inputs=+-
  Add7 : Sum
  Constant1 : Constant  Commented=on  Value=2*pi  OutDataTypeStr=single  SampleTime=-1
  Constant11 : Constant  Commented=on  Value=-pi  OutDataTypeStr=single  SampleTime=-1
  Constant12 : Constant  Value=pi  OutDataTypeStr=single  SampleTime=-1
  Constant13 : Constant  Value=-pi  OutDataTypeStr=single  SampleTime=-1
  Constant14 : Constant  Value=2*pi  OutDataTypeStr=single  SampleTime=-1
  Constant15 : Constant  Value=2*pi  OutDataTypeStr=single  SampleTime=-1
  Constant2 : Constant  Commented=on  Value=2*pi  OutDataTypeStr=single  SampleTime=-1
  Constant6 : Constant  Commented=on  Value=pi  OutDataTypeStr=single  SampleTime=-1
  Data Store Read1 : DataStoreRead  DataStoreName=oProp  DataStoreElements=oProp.oIsr_.oParam_.fControlLoopDt_  IndexOptions=Index vector (dialog)  Indices=1  OutputSizes=1
  Data Store Read29 : DataStoreRead  Commented=on  DataStoreName=oProp  DataStoreElements=oProp.oIsr_.oParam_.fControlLoopDt_  IndexOptions=Index vector (dialog)  Indices=1  OutputSizes=1
  Discrete-Time Integrator4 : DiscreteIntegrator  Commented=on  IntegratorMethod=Accumulation: Forward Euler  ExternalReset=rising  InitialConditionSource=external  SampleTime=-1  ShowStatePort=on  ICPrevOutput=DiscIntNeverNeededParam  ICPrevScaledInput=DiscIntNeverNeededParam
  Equal3 : RelationalOperator  Commented=on  Operator=>  OutDataTypeStr=boolean  RndMeth=Simplest
  Equal4 : RelationalOperator  Commented=on  Operator=<  OutDataTypeStr=boolean  RndMeth=Simplest
  Equal5 : RelationalOperator  Operator=>  OutDataTypeStr=boolean  RndMeth=Simplest
  Equal6 : RelationalOperator  Operator=<  OutDataTypeStr=boolean  RndMeth=Simplest
  Logical Operator : Logic  Commented=on  Operator=OR  AllPortsSameDT=off  OutDataTypeStr=boolean
  Logical Operator2 : Logic  Operator=OR  AllPortsSameDT=off  OutDataTypeStr=boolean
  Product1 : Product
  Product16 : Product  Commented=on
  Switch1 : Switch  Commented=on  Criteria=u2 > Threshold  Threshold=0.5
  Switch2 : Switch  Commented=on  Criteria=u2 > Threshold  Threshold=0.5
  Switch5 : Switch  Criteria=u2 > Threshold
  Switch6 : Switch  Criteria=u2 > Threshold  Threshold=0.5
  Switch7 : Switch  Criteria=u2 > Threshold  Threshold=0.5
  Unit Delay1 : UnitDelay  SampleTime=-1  HasFrameUpgradeWarning=on
  Angle : Outport
  wires:
  Switch6/1 -> Switch7/3
  Omega/1 -> Product1/1
  Switch7/1 -> Switch5/1
  Add5/1 -> Switch5/3, Equal5/1, Equal6/1, Add7/1, Add6/1, Switch6/3
  Constant12/1 -> Equal5/2
  Logical Operator2/1 -> Switch5/2
  Unit Delay1/1 -> Add5/1
  Constant15/1 -> Add7/2
  Equal6/1 -> Switch7/2, Logical Operator2/2
  Add6/1 -> Switch6/1
  Product1/1 -> Add5/2
  Data Store Read1/1 -> Product1/2
  Add7/1 -> Switch7/1
  Equal5/1 -> Switch6/2, Logical Operator2/1
  Switch5/1 -> Unit Delay1/1, Angle/1
  Constant13/1 -> Equal6/2
  Constant14/1 -> Add6/2
  Data Store Read29/1 -> Product16/2
  Add/1 -> Switch2/1
  Switch2/1 -> Switch1/3
  Add1/1 -> Switch1/1
  Constant2/1 -> Add1/2
  Constant1/1 -> Add/2
  Equal3/1 -> Switch2/2, Logical Operator/1
  Switch1/1 -> Discrete-Time Integrator4/3
  Constant11/1 -> Equal4/2
  Logical Operator/1 -> Discrete-Time Integrator4/2
  Constant6/1 -> Equal3/2
  Product16/1 -> Discrete-Time Integrator4/1
  Equal4/1 -> Switch1/2, Logical Operator/2
  Discrete-Time Integrator4/State -> Add1/1, Equal4/1, Add/1, Switch2/3, Equal3/1

== system Target_Control_System/Target_Control_System/InterruptFunction/propMotor_isrTask/abcToAlphaBeta/ModelSourceFOProp ==
  note: 1) Add Subsystem or Model blocks as valid variant choices.
      | 2) You cannot connect blocks at this level. At simulation, connectivity is automatically
      | determined, based on the active variant and port name matching.
  DoNotIncludeCustomCode : Subsystem  TreatAsAtomicUnit=on  VariantControl=TARGET_CODE_GEN == 0
  IncludeCustomCode : Subsystem  TreatAsAtomicUnit=on  VariantControl=(default)

== system Target_Control_System/Target_Control_System/InterruptFunction/propMotor_isrTask/abcToAlphaBeta/vsincos() ==
  Input : Inport  OutDataTypeStr=single
  Input1 : Inport  Port=2  OutDataTypeStr=single
  Enable : EnablePort
  Cos : Trigonometry  Operator=cos
  Cos1 : Trigonometry  Operator=cos
  Data Store Write : DataStoreWrite  DataStoreName=mdl_fUphFilterDelayAngleRad_cos_  IndexOptions=Index vector (dialog)  Indices=1  OutputSizes=1
  Data Store Write10 : DataStoreWrite  DataStoreName=mdl_fFluxMainAngleRaw2_sin_  IndexOptions=Index vector (dialog)  Indices=1  OutputSizes=1
  Data Store Write11 : DataStoreWrite  DataStoreName=mdl_fFluxMainAngleRaw2_cos_  IndexOptions=Index vector (dialog)  Indices=1  OutputSizes=1
  Data Store Write6 : DataStoreWrite  DataStoreName=mdl_fUphFilterDelayAngleRad_sin_  IndexOptions=Index vector (dialog)  Indices=1  OutputSizes=1
  Sin : Trigonometry
  Sin1 : Trigonometry
  wires:
  Input/1 -> Sin/1, Cos/1
  Cos/1 -> Data Store Write/1
  Input1/1 -> Sin1/1, Cos1/1
  Sin1/1 -> Data Store Write10/1
  Sin/1 -> Data Store Write6/1
  Cos1/1 -> Data Store Write11/1
